simulink model "Sim_EPSw"  (R2020b)
settings: Solver=VariableStepAuto  StartTime=0.0  StopTime=8  MaxStep=1e-3  RelTol=1e-3
values from neighbouring files (symbols this model uses):
  Amplitude = 4    [Sim_Paras_Init.m]
  Cc = 5    [Sim_Paras_Init.m]
  Cd = 0.2    [Sim_Paras_Init.m]
  Cm = 0.034    [Sim_Paras_Init.m]
  Cr = 210    [Sim_Paras_Init.m]
  Input_Fre = (0.5)*2*pi    (= 3.14159265359)    [Sim_Paras_Init.m]
  Jc = 0.06    [Sim_Paras_Init.m]
  Jd = 0.04    [Sim_Paras_Init.m]
  Jm = 0.016    [Sim_Paras_Init.m]
  KD = 3    [Sim_Paras_Init.m]
  Kd = 10    [Sim_Paras_Init.m]
  Ke = 3    [Sim_Paras_Init.m]
  Ki = 5    [Sim_Paras_Init.m]
  Km = 130    [Sim_Paras_Init.m]
  Kp = 10    [Sim_Paras_Init.m]
  Kr = 13852    [Sim_Paras_Init.m]
  Ks = 150    [Sim_Paras_Init.m]
  mr = 2.5    [Sim_Paras_Init.m]
  N = 20    [Sim_Paras_Init.m]
  Rad2deg = 1/2/pi*360    (= 57.2957795131)    [Sim_Paras_Init.m]
  rp = 0.008    [Sim_Paras_Init.m]
  Sin_flag = 1    [Sim_Paras_Init.m]
  tau1 = 0.1    [Sim_Paras_Init.m]
  tau2 = 0.08    [Sim_Paras_Init.m]
settings Model: Creator=Administrator  LastModifiedBy=Administrator
settings DataIOCC: ReturnWorkspaceOutputs=off

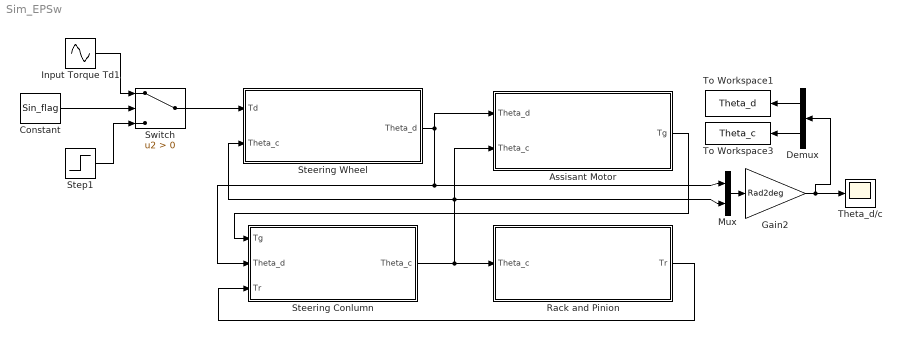
== system Sim_EPSw ==
  Assisant Motor : Subsystem
  Constant : Constant  Value=Sin_flag
  Demux : Demux  Outputs=2
  Gain2 : Gain  Gain=Rad2deg
  Input Torque Td1 : Sin  Amplitude=Amplitude  Frequency=Input_Fre  SampleTime=0
  Mux : Mux  Inputs=2
  Rack and Pinion : Subsystem
  Steering Conlumn : Subsystem
  Steering Wheel : Subsystem
  Step1 : Step  Time=0  After=Amplitude  SampleTime=0
  Switch : Switch  Criteria=u2 > Threshold
  Theta_d/c : Scope
  To Workspace1 : ToWorkspace  VariableName=Theta_d  SaveFormat=Timeseries  SampleTime=-1
  To Workspace3 : ToWorkspace  VariableName=Theta_c  SaveFormat=Timeseries  SampleTime=-1
  wires:
  Steering Conlumn/1(Theta_c) -> Rack and Pinion/1(Theta_c), Mux/2, Assisant Motor/2(Theta_c), Steering Wheel/2(Theta_c)
  Assisant Motor/1(Tg) -> Steering Conlumn/1(Tg)
  Rack and Pinion/1(Tr) -> Steering Conlumn/3(Tr)
  Gain2/1 -> Demux/1, Theta_d/c/1
  Steering Wheel/1(Theta_d) -> Steering Conlumn/2(Theta_d), Mux/1, Assisant Motor/1(Theta_d)
  Mux/1 -> Gain2/1
  Demux/1 -> To Workspace1/1
  Demux/2 -> To Workspace3/1
  Switch/1 -> Steering Wheel/1(Td)
  Constant/1 -> Switch/2
  Input Torque Td1/1 -> Switch/1
  Step1/1 -> Switch/3

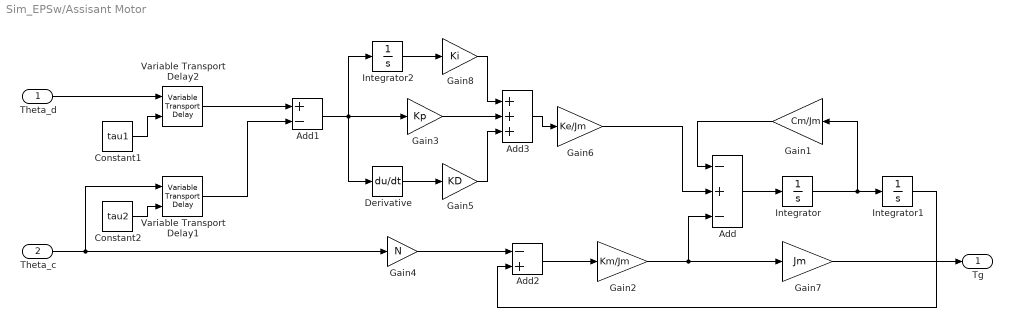
== system Sim_EPSw/Assisant Motor ==
  Theta_d : Inport
  Theta_c : Inport  Port=2
  Add : Sum  Inputs=-+-
  Add1 : Sum  Inputs=+-
  Add2 : Sum  Inputs=-+
  Add3 : Sum  Inputs=+++
  Constant1 : Constant  Value=tau1
  Constant2 : Constant  Value=tau2
  Derivative : Derivative
  Gain1 : Gain  Gain=Cm/Jm
  Gain2 : Gain  Gain=Km/Jm
  Gain3 : Gain  Gain=Kp
  Gain4 : Gain  Gain=N
  Gain5 : Gain  Gain=KD
  Gain6 : Gain  Gain=Ke/Jm
  Gain7 : Gain  Gain=Jm
  Gain8 : Gain  Gain=Ki
  Integrator : Integrator
  Integrator1 : Integrator
  Integrator2 : Integrator
  Variable Transport Delay1 : VariableTransportDelay  VariableDelayType=Variable transport delay  MaximumDelay=10
  Variable Transport Delay2 : VariableTransportDelay  VariableDelayType=Variable transport delay  MaximumDelay=10
  Tg : Outport
  wires:
  Gain2/1 -> Gain7/1, Add/3
  Add2/1 -> Gain2/1
  Theta_c/1 -> Variable Transport Delay1/1, Gain4/1
  Gain1/1 -> Add/1
  Integrator1/1 -> Add2/2
  Integrator/1 -> Integrator1/1, Gain1/1
  Add/1 -> Integrator/1
  Gain4/1 -> Add2/1
  Add1/1 -> Integrator2/1, Derivative/1, Gain3/1
  Derivative/1 -> Gain5/1
  Gain3/1 -> Add3/2
  Gain5/1 -> Add3/3
  Add3/1 -> Gain6/1
  Gain7/1 -> Tg/1
  Integrator2/1 -> Gain8/1
  Gain8/1 -> Add3/1
  Gain6/1 -> Add/2
  Constant1/1 -> Variable Transport Delay2/2
  Constant2/1 -> Variable Transport Delay1/2
  Theta_d/1 -> Variable Transport Delay2/1
  Variable Transport Delay2/1 -> Add1/1
  Variable Transport Delay1/1 -> Add1/2

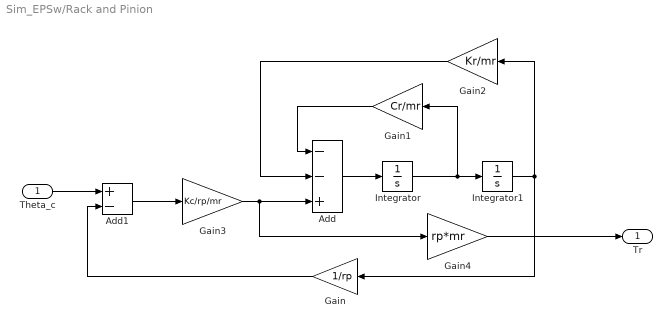
== system Sim_EPSw/Rack and Pinion ==
  Theta_c : Inport
  Add : Sum  Inputs=--+
  Add1 : Sum  Inputs=+-
  Gain : Gain  Gain=1/rp
  Gain1 : Gain  Gain=Cr/mr
  Gain2 : Gain  Gain=Kr/mr
  Gain3 : Gain  Gain=Kc/rp/mr
  Gain4 : Gain  Gain=rp*mr
  Integrator : Integrator
  Integrator1 : Integrator
  Tr : Outport
  wires:
  Gain2/1 -> Add/2
  Add/1 -> Integrator/1
  Integrator/1 -> Gain1/1, Integrator1/1
  Integrator1/1 -> Gain/1, Gain2/1
  Gain1/1 -> Add/1
  Theta_c/1 -> Add1/1
  Gain3/1 -> Gain4/1, Add/3
  Gain/1 -> Add1/2
  Add1/1 -> Gain3/1
  Gain4/1 -> Tr/1

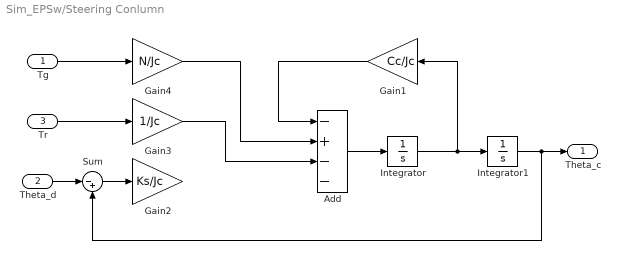
== system Sim_EPSw/Steering Conlumn ==
  Tg : Inport
  Theta_d : Inport  Port=2
  Tr : Inport  Port=3
  Add : Sum  Inputs=-+--
  Gain1 : Gain  Gain=Cc/Jc
  Gain2 : Gain  Gain=Ks/Jc
  Gain3 : Gain  Gain=1/Jc
  Gain4 : Gain  Gain=N/Jc
  Integrator : Integrator
  Integrator1 : Integrator
  Sum : Sum  Inputs=|-+
  Theta_c : Outport
  wires:
  Add/1 -> Integrator/1
  Integrator/1 -> Integrator1/1, Gain1/1
  Integrator1/1 -> Theta_c/1, Sum/2
  Tg/1 -> Gain4/1
  Gain4/1 -> Add/2
  Theta_d/1 -> Sum/1
  Sum/1 -> Gain2/1
  Gain1/1 -> Add/1
  Tr/1 -> Gain3/1
  Gain3/1 -> Add/3

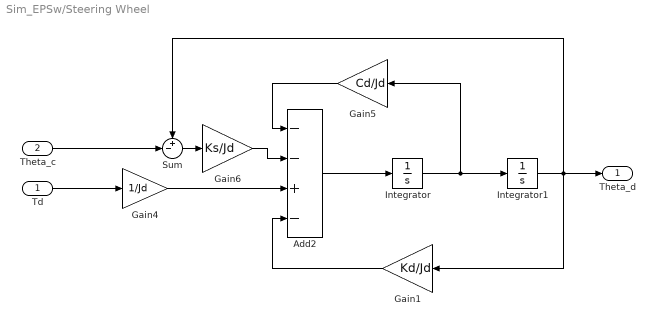
== system Sim_EPSw/Steering Wheel ==
  Td : Inport
  Theta_c : Inport  Port=2
  Add2 : Sum  Inputs=--+-
  Gain1 : Gain  Gain=Kd/Jd
  Gain4 : Gain  Gain=1/Jd
  Gain5 : Gain  Gain=Cd/Jd
  Gain6 : Gain  Gain=Ks/Jd
  Integrator : Integrator
  Integrator1 : Integrator
  Sum : Sum  Inputs=+-|
  Theta_d : Outport
  wires:
  Integrator/1 -> Gain5/1, Integrator1/1
  Add2/1 -> Integrator/1
  Td/1 -> Gain4/1
  Gain4/1 -> Add2/3
  Gain5/1 -> Add2/1
  Integrator1/1 -> Gain1/1, Sum/1, Theta_d/1
  Sum/1 -> Gain6/1
  Gain6/1 -> Add2/2
  Theta_c/1 -> Sum/2
  Gain1/1 -> Add2/4
